simulink model "CruiseControl_Perfect_TestHarness"  (R2020a)
settings: configuration reference "ModelReferencingVisual" (kept outside this file)
libraries: SignalEditorBlockLib x1
settings Model: DataDictionary=CruiseControl_Req_dd.sldd  Creator=colosky  LastModifiedBy=promero
settings ConfigSetRef: SourceName=ModelReferencingVisual

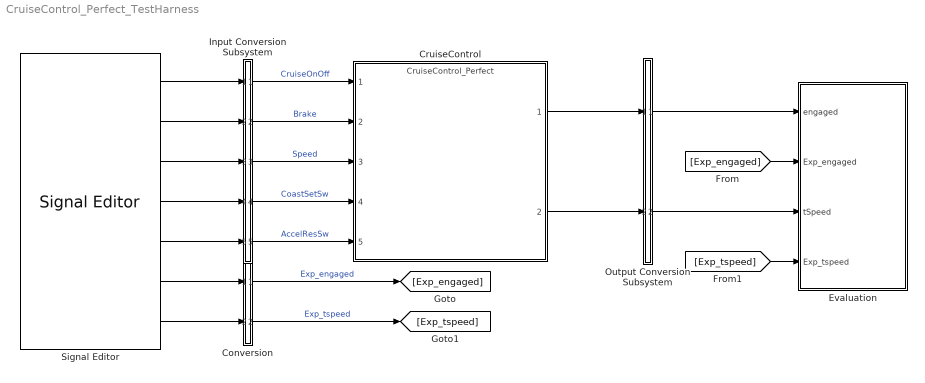
== system CruiseControl_Perfect_TestHarness ==
  Conversion : Subsystem
      mask Display: disp('');
  CruiseControl : ModelReference  ModelNameDialog=CruiseControl_Perfect  SimulationMode=Normal  CodeInterface=Top model  ModelReferenceVersion=1.470
  Evaluation : Subsystem
  Input Conversion Subsystem : Subsystem  Tag=__SLT_ICS__
  Output Conversion Subsystem : Subsystem  Tag=__SLT_OCS__
  Signal Editor : SignalEditorBlockLib/Signal Editor  FileName=TestInputs.mat  ActiveScenario=Engage_AccelResSw_Veh_Spd  ActiveSignal=Exp_tspeed  IsBus=off  OutputBusObjectStr=Bus: BusObject  SampleTime=0  OutputAfterFinalValue=Extrapolation  Unit=inherit  PreserveSignalName=on
  wires:
  Signal Editor/1 -> Input Conversion Subsystem/1(In_1)
  Signal Editor/2 -> Input Conversion Subsystem/2(In_2)
  Signal Editor/3 -> Input Conversion Subsystem/3(In_3)
  Signal Editor/4 -> Input Conversion Subsystem/4(In_4)
  Signal Editor/5 -> Input Conversion Subsystem/5(In_5)
  Input Conversion Subsystem/1(Out_1) -> CruiseControl/1  "CruiseOnOff"
  Input Conversion Subsystem/2(Out_2) -> CruiseControl/2  "Brake"
  Input Conversion Subsystem/3(Out_3) -> CruiseControl/3  "Speed"
  Input Conversion Subsystem/4(Out_4) -> CruiseControl/4  "CoastSetSw"
  Input Conversion Subsystem/5(Out_5) -> CruiseControl/5  "AccelResSw"
  CruiseControl/1 -> Output Conversion Subsystem/1(In_1)
  CruiseControl/2 -> Output Conversion Subsystem/2(In_2)
  Signal Editor/6 -> Conversion/1(In6)
  Signal Editor/7 -> Conversion/2(In7)
  Conversion/1(Out6) -> [Exp_engaged]  "Exp_engaged"
  Conversion/2(Out7) -> [Exp_tspeed]  "Exp_tspeed"
  Output Conversion Subsystem/1(Out_1) -> Evaluation/1(engaged)
  Output Conversion Subsystem/2(Out_2) -> Evaluation/3(tSpeed)
  [Exp_engaged] -> Evaluation/2(Exp_engaged)
  [Exp_tspeed] -> Evaluation/4(Exp_tspeed)

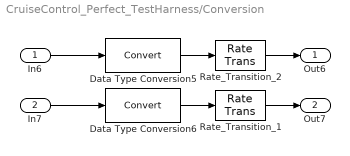
== system CruiseControl_Perfect_TestHarness/Conversion ==
  In6 : Inport
  In7 : Inport  Port=2
  Data Type Conversion5 : DataTypeConversion
  Data Type Conversion6 : DataTypeConversion
  Rate_Transition_1 : RateTransition  OutPortSampleTime=0.1
  Rate_Transition_2 : RateTransition  OutPortSampleTime=0.1
  Out6 : Outport  VectorParamsAs1DForOutWhenUnconnected=off
  Out7 : Outport  Port=2  VectorParamsAs1DForOutWhenUnconnected=off
  wires:
  Data Type Conversion5/1 -> Rate_Transition_2/1
  In6/1 -> Data Type Conversion5/1
  Data Type Conversion6/1 -> Rate_Transition_1/1
  In7/1 -> Data Type Conversion6/1
  Rate_Transition_2/1 -> Out6/1
  Rate_Transition_1/1 -> Out7/1

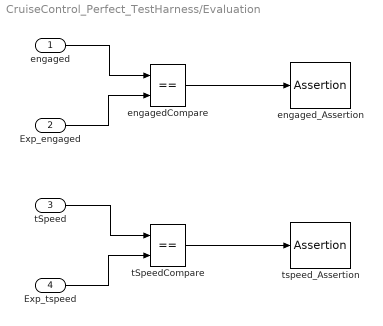
== system CruiseControl_Perfect_TestHarness/Evaluation ==
  engaged : Inport
  Exp_engaged : Inport  Port=2
  tSpeed : Inport  Port=3
  Exp_tspeed : Inport  Port=4
  engagedCompare : RelationalOperator  Operator===  OutDataTypeStr=boolean  RndMeth=Nearest  InputSameDT=on
  engaged_Assertion : Assertion  StopWhenAssertionFail=off
  tSpeedCompare : RelationalOperator  Operator===  OutDataTypeStr=boolean  RndMeth=Nearest  InputSameDT=on
  tspeed_Assertion : Assertion  StopWhenAssertionFail=off
  wires:
  Exp_engaged/1 -> engagedCompare/2
  engaged/1 -> engagedCompare/1
  Exp_tspeed/1 -> tSpeedCompare/2
  tSpeed/1 -> tSpeedCompare/1
  engagedCompare/1 -> engaged_Assertion/1
  tSpeedCompare/1 -> tspeed_Assertion/1

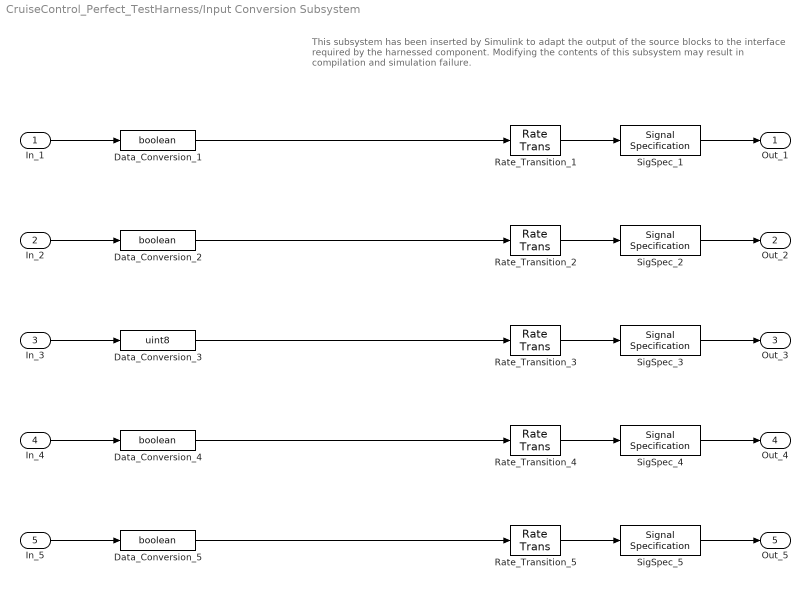
== system CruiseControl_Perfect_TestHarness/Input Conversion Subsystem ==
  note: This subsystem has been inserted by Simulink to adapt the output of the source blocks to the interface required by the harnessed component.
      |  Modifying the contents of this subsystem may result in compilation and simulation failure.
  In_1 : Inport
  In_2 : Inport  Port=2
  In_3 : Inport  Port=3
  In_4 : Inport  Port=4
  In_5 : Inport  Port=5
  Data_Conversion_{1..2,4..5} (4 alike) : DataTypeConversion  OutDataTypeStr=boolean  SaturateOnIntegerOverflow=on  RndMeth=Zero
  Data_Conversion_3 : DataTypeConversion  OutDataTypeStr=uint8  SaturateOnIntegerOverflow=on  RndMeth=Zero
  Rate_Transition_{1..5} (5 alike) : RateTransition  OutPortSampleTime=0.1
  SigSpec_{1..2,4..5} (4 alike) : SignalSpecification  OutDataTypeStr=boolean  Dimensions=[1]  SampleTime=0.1
  SigSpec_3 : SignalSpecification  OutDataTypeStr=uint8  Dimensions=[1]  SampleTime=0.1
  Out_1 : Outport  VectorParamsAs1DForOutWhenUnconnected=off
  Out_2 : Outport  Port=2  VectorParamsAs1DForOutWhenUnconnected=off
  Out_3 : Outport  Port=3  VectorParamsAs1DForOutWhenUnconnected=off
  Out_4 : Outport  Port=4  VectorParamsAs1DForOutWhenUnconnected=off
  Out_5 : Outport  Port=5  VectorParamsAs1DForOutWhenUnconnected=off
  wires:
  In_1/1 -> Data_Conversion_1/1
  Data_Conversion_1/1 -> Rate_Transition_1/1
  In_2/1 -> Data_Conversion_2/1
  Data_Conversion_2/1 -> Rate_Transition_2/1
  In_3/1 -> Data_Conversion_3/1
  Data_Conversion_3/1 -> Rate_Transition_3/1
  In_4/1 -> Data_Conversion_4/1
  Data_Conversion_4/1 -> Rate_Transition_4/1
  In_5/1 -> Data_Conversion_5/1
  Data_Conversion_5/1 -> Rate_Transition_5/1
  Rate_Transition_1/1 -> SigSpec_1/1
  Rate_Transition_2/1 -> SigSpec_2/1
  Rate_Transition_3/1 -> SigSpec_3/1
  Rate_Transition_4/1 -> SigSpec_4/1
  Rate_Transition_5/1 -> SigSpec_5/1
  SigSpec_1/1 -> Out_1/1
  SigSpec_2/1 -> Out_2/1
  SigSpec_3/1 -> Out_3/1
  SigSpec_4/1 -> Out_4/1
  SigSpec_5/1 -> Out_5/1

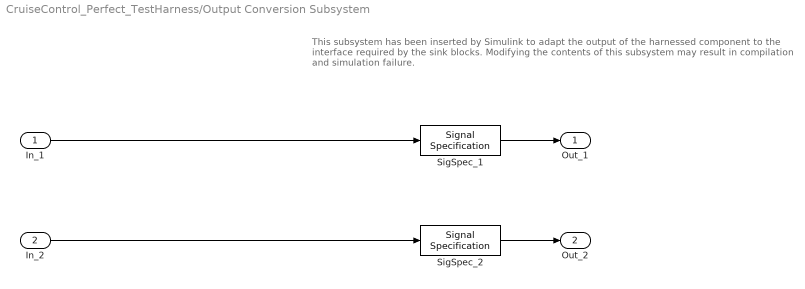
== system CruiseControl_Perfect_TestHarness/Output Conversion Subsystem ==
  note: This subsystem has been inserted by Simulink to adapt the output of the harnessed component to the interface required by the sink blocks.
      |  Modifying the contents of this subsystem may result in compilation and simulation failure.
  In_1 : Inport
  In_2 : Inport  Port=2
  SigSpec_1 : SignalSpecification  OutDataTypeStr=boolean  Dimensions=[1]  SampleTime=0.1
  SigSpec_2 : SignalSpecification  OutDataTypeStr=uint8  Dimensions=[1]  SampleTime=0.1
  Out_1 : Outport  VectorParamsAs1DForOutWhenUnconnected=off
  Out_2 : Outport  Port=2  VectorParamsAs1DForOutWhenUnconnected=off
  wires:
  SigSpec_1/1 -> Out_1/1
  SigSpec_2/1 -> Out_2/1
  In_1/1 -> SigSpec_1/1
  In_2/1 -> SigSpec_2/1
